simulink model "Example_3_Open"  (Simulink 8.3)
settings: Solver=ode45  StartTime=0.0  StopTime=50  RelTol=1e-3
settings Model: Creator=NeuControl  LastModifiedBy=Li Jinghao
settings DataIOCC: SignalLoggingSaveFormat=Dataset
settings DebuggingCC: UnderspecifiedInitializationDetection=Simplified  StateNameClashWarn=none
settings GRTTargetCC: CombineOutputUpdateFcns=on  GRTInterface=off

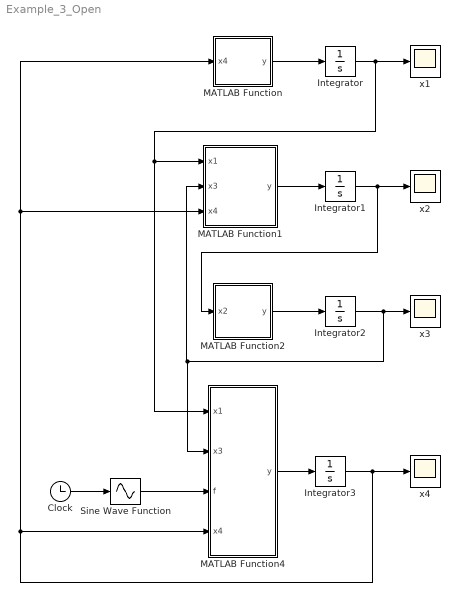
== system Example_3_Open ==
  Clock : Clock
  Integrator : Integrator  InitialCondition=pi/6
  Integrator1 : Integrator
  Integrator2 : Integrator
  Integrator3 : Integrator
  MATLAB Function : MATLAB Function  TreatAsAtomicUnit=on
  MATLAB Function1 : MATLAB Function  TreatAsAtomicUnit=on
  MATLAB Function2 : MATLAB Function  TreatAsAtomicUnit=on
  MATLAB Function4 : MATLAB Function  TreatAsAtomicUnit=on
  Sine Wave Function : Sin  TimeSource=Use external signal  SampleTime=0
  x{1..4} (4 alike) : Scope
      x1 settings: SaveName=x1
      x2 settings: SaveName=x2
      x3 settings: SaveName=x3
      x4 settings: SaveName=x4
  wires:
  Integrator/1 -> MATLAB Function4/1(x1), MATLAB Function1/1(x1), x1/1
  MATLAB Function/1(y) -> Integrator/1
  MATLAB Function1/1(y) -> Integrator1/1
  Integrator1/1 -> MATLAB Function2/1(x2), x2/1
  Integrator2/1 -> MATLAB Function4/2(x3), MATLAB Function1/2(x3), x3/1
  MATLAB Function2/1(y) -> Integrator2/1
  MATLAB Function4/1(y) -> Integrator3/1
  Integrator3/1 -> x4/1, MATLAB Function/1(x4), MATLAB Function1/3(x4), MATLAB Function4/4(x4)
  Sine Wave Function/1 -> MATLAB Function4/3(f)
  Clock/1 -> Sine Wave Function/1

== matlab function MATLAB Function1 ==
  data: x1 input double; x3 input double; x4 input double; y output double
function y = fcn(x1,x3,x4)
%#codegen

m=2;
M=8;
l=0.5;

y = x3-m*l/(m+M)*cos(x1)*x4;

== matlab function MATLAB Function ==
  data: x4 input double; y output double
function y = fcn(x4)
%#codegen

y = x4;

== matlab function MATLAB Function2 ==
  data: x2 input double; y output double
function y = fcn(x2)
%#codegen

m=2;
M=8;
k=0.5;
y = -k/(m+M)*x2;

== matlab function MATLAB Function4 ==
  data: x1 input double; x3 input double; f input double; x4 input double; y output double
function y = fcn(x1,x3,f,x4)
%#codegen

m=2;
M=8;
l=0.5;
k=0.5;
y = 1/(4/3*m*l*l*(m+M)-m*m*l*l*cos(x1)*cos(x1))...
    *(-m*m*l*l*sin(x1)*cos(x1)*x4+k*m*l*cos(x1)*x3+(m+M)*f);
